simulink model "CONTROL_02"  (R2018b)
settings: Solver=FixedStepAuto  StartTime=0.0  StopTime=10  FixedStep=0.01  RelTol=1e-3
model workspace: external: MATLAB File D:\OneDrive\STUDY\RIC LAB\PROJECT 6DOF\CODE\CODE 6DOF\07_CONTROL\CONTROL_02\ROBOT_DataFile.m (data not in the file)
values from neighbouring files (symbols this model uses):
  k1 = [k11 k12 k13 k14 k15 k16]    [GA_CTC_01.m]
  k2 = [k21 k22 k23 k24 k25 k26]    [GA_CTC_01.m]
undefined symbols (not defined in the file or in its folder): smiData, X, Y, Z
libraries: sm_lib x35, nesl_utility x7
(part 14 of 14)

== matlab function CONTROL_02/Data ==
  data: m output; L output; Pic output; I output
function [m,L,Pic,I] = DATA_6DOF()
a1=0.075; a2=0.270; a3=0.090; d1=0.335; d4=0.295; d7=0.08;
m1 = 5.6511; m2 = 4.6061; m3 = 4.2963; m4 = 1.9151; m5 = 0.3399; m6 = 0.0714;
m = [m1 m2 m3 m4 m5 m6];
L = [a1 a2 a3 d1 d4 d7];
% Pic = zeros(6,3);
% I = zeros(6,6);
Pic = [0.0373,  -0.0076,   0.1064;
       0.1127,   0.0065,   0.0648;
       0.0447,   0.0125,  -0.0554;
       0.0006,   0.0052,   0.1068;
            0,   0.0062,   0.0195;
     -0.00001,  0.00001,  0.01126];

% I1 = [ 0.0320,  -0.0017,   0.0093;
%       -0.0017,   0.0364,  -0.0018;
%        0.0093,  -0.0018,   0.0334];
I1 = [0.0320, 0.0364, 0.0334, 0.0017, 0.0018, -0.0093];
% I2 = [ 0.0099,   0.0008,  -0.0002;
%        0.0008,   0.0646,   0.0002;
%       -0.0002,   0.0002,   0.0684];
I2 = [0.0099, 0.0646, 0.0684, -0.0008, -0.0002, 0.0002];
% I3 = [ 0.0176,    0.001,   0.0007;
%         0.001,   0.0195,   0.0002;
%        0.0007,   0.0002,    0.024];
I3 = [0.0176, 0.0195, 0.024, -0.001, -0.0002, -0.0007];
% I4 =  [  0.009,        0,        0;
%              0,   0.0081,   0.0002;
%              0,   0.0002,   0.0037];
I4 = [0.009, 0.0081, 0.0037, -0, -0.0002, -0];
% I5 = [ 0.0003,        0,        0;
%             0,   0.0002,        0;
%             0,        0,   0.0003];
I5 = [0.0003, 0.0002, 0.0003, 0, 0, 0];
% I6 = [ 0.00002,        0,        0;
%              0,  0.00002,        0;
%              0,        0,  0.00003];
I6 = [0.00002, 0.0002, 0.0003, 0, 0, 0];
I = [I1; I2; I3; I4; I5; I6];

== matlab function CONTROL_02/Computed Torque Control ==
  data: the input; dthe input; the_r input; to output; dthe_r input; ddthe_r input; M input; C input; G input; E output
function [to,E] = CTC(the,dthe,the_r,dthe_r,ddthe_r,M,C,G)
%% Control:
% Controler parameters
% GA
% k1 65.7400   52.0100   59.6700   97.0800    3.1400   41.8200
% k2 98.7800   88.4900   62.1600   67.4800   71.0500   35.0600
% k11 = k1(1); k12 = k1(2); k13 = k1(3); k14 = k1(4); k15 = k1(5); k16 = k1(6);
% k21 = k2(1); k22 = k2(2); k23 = k2(3); k24 = k2(4); k25 = k2(5); k26 = k2(6);
% Kp = diag([k11,k12,k13,k14,k15,k16]);
% Kv = diag([k21,k22,k23,k24,k25,k26]);
% CTC
ld1 = 10;
ld2 = 10;
ld3 = 10;
ld4 = 28;
ld5 = 65;
ld6 = 80;
Kp = diag([ld1^2,ld2^2,ld3^2,ld4^2,ld5^2,ld6^2]);
Kv = 2*diag([ld1,ld2,ld3,ld4,ld5,ld6]);

% Designed computed torque control
E = the_r - the;
dE = dthe_r - dthe;
alpha = M;
beta = C*dthe + G;
dto = ddthe_r + Kv*dE + Kp*E;
to = alpha*dto + beta;

== matlab function CONTROL_02/MATLAB Function ==
  data: u input; y output
function y = fcn(u)

if u >=10 && u<10.1
    y = 100;
elseif u >=13 && u<13.1
    y = -50;
else
    y = 0;
end

== matlab function CONTROL_02/MATLAB Function1 ==
  data: u input; y output
function y = fcn(u)

if u >=20 && u<20.1
    y = 250;
elseif u >=23 && u<23.1
    y = -250;
else
    y = 0;
end

== matlab function CONTROL_02/MATLAB Function2 ==
  data: u input; y output
function y = fcn(u)

if u >= 3 && u < 3.1
    y = 300;
elseif u >= 6 && u < 6.1
    y = -300;
else
    y = 0;
end

== matlab function CONTROL_02/Sliding Mode Control ==
  data: the input; dthe input; the_r input; to output; dthe_r input; ddthe_r input; M input; C input; G input; s output; e_d output
function [to,s,e_d] = SMC(the,dthe,the_r,dthe_r,ddthe_r,M,C,G)
%% Control:
% Controler parameters
% % with noise

% without noise
lamda = 50*diag([1,1,1,1,1,1]);
K     = 0.055*diag([1,1,1,1,1,1]);
eta   = 0.1*diag([1,1,1,1,1,1]);

% Designed sliding mode control
e = the - the_r;
e_d = dthe - dthe_r;
s = lamda*e + e_d;
to = -K*s + C*(dthe_r - lamda*e) + G + M*(ddthe_r - lamda*e_d) - eta*sign(s);
% to = -K*s + C*(dthe_r - lamda*e) + G + M*(ddthe_r - lamda*e_d) - eta*min(0.1, max(-0.1, s));

== matlab function CONTROL_02/Adaptive Sliding Mode Control ==
  data: the input; dthe input; the_r input; to output; dthe_r input; ddthe_r input; M input; C input; G input; s output; e_d output; eta_hat input; etad_hat output
function [to,s,e_d,etad_hat] = ASMC(the,dthe,the_r,dthe_r,ddthe_r,M,C,G,eta_hat)
%% Control:
% Controler parameters
% % with noise

% without noise
lamda = diag([20,20,20,20,20,20]);
K = diag([5,5,5,5,5,5]);
k1 = 10^-2*[3;3;2;0.5;0.2;0.1];
k2 = 10^-4*[500;300;200;100;100;100];

% Designed sliding mode control
e = the - the_r;
e_d = dthe - dthe_r;
s = e_d + lamda*e;

e_2 = 0.001;
e_1 = 10*e_2;
etm = zeros(6,1);
for i = 1:6
    gamma = sign(abs(s(i)) - e_1);
    if     (min(abs(s(i))) >= e_2 && eta_hat(i,i) > 0)
        etm(i) = k1(i)*((k2(i)^-1*(abs(s(i))))^gamma)*gamma;
    elseif (min(abs(s(i))) >= e_2 && eta_hat(i,i) == 0)
        etm(i) = k1(i)*k2(i)*(abs(s(i)))^-1;
    else
        etm(i) = 0;
    end
end
etad_hat = diag(etm);

to = -K*s + C*(dthe_r - lamda*e) + G + M*(ddthe_r - lamda*e_d) - eta_hat*sign(s);
% to = -K*s + C*(dthe_r - lamda*e) + G + M*(ddthe_r - lamda*e_d) - eta_hat*min(0.1, max(-0.1, s));
%%
% k=      diag([7.61,3.3]);
% lamda=  diag([77.54,75.76]);
% 
% e=theta-theta_i;
% e_d = theta_d - theta_i_d;
% s = e_d+lamda*e;
% 
% if (abs(s(1))>0.5)
%     eta_d1= k11*abs(s(1));
% else
%     eta_d1=-k21*abs(s(1));
% end
% 
% if (abs(s(2))>0.5)
%     eta_d2= k12*abs(s(2));
% else
%     eta_d2=-k22*abs(s(2));
% end
% 
% eta_d= [eta_d1,eta_d2]';
% 
% u= -k*s+C*(theta_i_d-lamda*e)+G+M*(theta_i_dd-lamda*e_d)-diag(eta)*sign(s);

== matlab function CONTROL_02/PID Control/PID ==
  data: e input; ei input; to output; ed input
function to = fcn(e,ei,ed)
Kp = 20*diag([1,1,1,1,1,1]);
Ki = 0*diag([1,1,1,1,1,1]);
Kd = 0.01*diag([1,1,1,1,1,1]);
to = Kp*e + Ki*ei + Kd*ed;

== matlab function CONTROL_02/Extended State Observer ==
  data: dt_ESO output; k0 input; to input; x1 input; M input; C input; G input; dx_hat output; x_hat input; x3_hat output
function [dt_ESO,dx_hat,x3_hat] = ESO(k0,to,x1,M,C,G,x_hat)
x1_hat = [x_hat(1);   x_hat(2);  x_hat(3);  x_hat(4);  x_hat(5);  x_hat(6)];
x2_hat = [x_hat(7);   x_hat(8);  x_hat(9); x_hat(10); x_hat(11); x_hat(12)];
x3_hat = [x_hat(13); x_hat(14); x_hat(15); x_hat(16); x_hat(17); x_hat(18)];
An = [zeros(6)   eye(6) zeros(6);
      zeros(6) zeros(6)   eye(6);
      zeros(6) zeros(6) zeros(6)]; %18x18
H = inv(M);                        %6x6
Bn = [zeros(6); H; zeros(6)];      %18x6
F = -inv(M)*(C*x2_hat + G);        %6x1
phi = [zeros(6,1); F; zeros(6,1)]; %18x1
K = [diag([  3*k0,  3*k0,  3*k0,  3*k0,  3*k0,  3*k0]);
     diag([3*k0^2,3*k0^2,3*k0^2,3*k0^2,3*k0^2,3*k0^2]);
     diag([  k0^3,  k0^3,  k0^3,  k0^3,  k0^3,  k0^3])]; %18x6
dx_hat = An*x_hat + Bn*to +  phi + K*(x1 - x1_hat);
dt_ESO = - M*x3_hat;

== matlab function CONTROL_02/SMC ESO ==
  data: the input; dthe input; the_r input; to output; dthe_r input; ddthe_r input; M input; C input; G input; s output; e_d output
function [to,s,e_d] = SMC(the,dthe,the_r,dthe_r,ddthe_r,M,C,G)
%% Control:
% Controler parameters
% % with noise

% without noise
lamda = 50*diag([1,1,1,1,1,1]);
K     = 0.055*diag([1,1,1,1,1,1]);
eta   = 0.1*diag([1,1,1,1,1,1]);

% Designed sliding mode control
e = the - the_r;
e_d = dthe - dthe_r;
s = lamda*e + e_d;
to = -K*s + C*(dthe_r - lamda*e) + G + M*(ddthe_r - lamda*e_d) - eta*sign(s);
% to = -K*s + C*(dthe_r - lamda*e) + G + M*(ddthe_r - lamda*e_d) - eta*min(0.1, max(-0.1, s));
